simulink model "MdXXHolderChk"  (R2024b)
settings: Solver=FixedStepDiscrete  StartTime=0.0  StopTime=10.0  FixedStep=0.01  RelTol=1e-3
undefined symbols (not defined in the file or in its folder): KeSMSwAcsMd32SecRwLtStBkReclnUpwdDnwdPos1_Val, KeSMSwAcsMd53SecRwRtStBkReclnUpwdDnwdPos1_Val, SeatChldLkSt
libraries: simulink x41
(part 3 of 5)

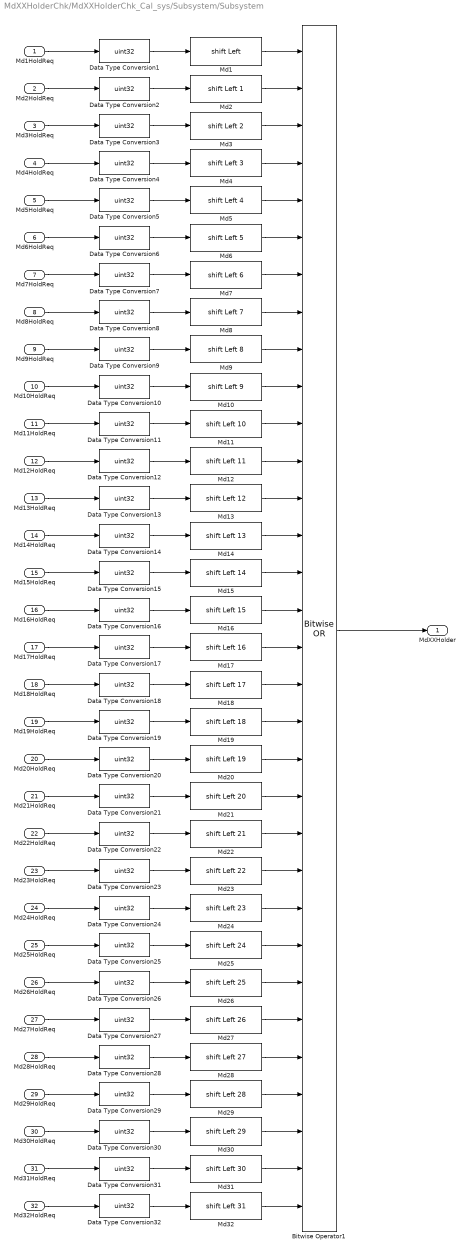
== system MdXXHolderChk/MdXXHolderChk_Cal_sys/Subsystem/Subsystem ==
  Md1HoldReq : Inport
  Md2HoldReq : Inport  Port=2
  Md3HoldReq : Inport  Port=3
  Md4HoldReq : Inport  Port=4
  Md5HoldReq : Inport  Port=5
  Md6HoldReq : Inport  Port=6
  Md7HoldReq : Inport  Port=7
  Md8HoldReq : Inport  Port=8
  Md9HoldReq : Inport  Port=9
  Md10HoldReq : Inport  Port=10
  Md11HoldReq : Inport  Port=11
  Md12HoldReq : Inport  Port=12
  Md13HoldReq : Inport  Port=13
  Md14HoldReq : Inport  Port=14
  Md15HoldReq : Inport  Port=15
  Md16HoldReq : Inport  Port=16
  Md17HoldReq : Inport  Port=17
  Md18HoldReq : Inport  Port=18
  Md19HoldReq : Inport  Port=19
  Md20HoldReq : Inport  Port=20
  Md21HoldReq : Inport  Port=21
  Md22HoldReq : Inport  Port=22
  Md23HoldReq : Inport  Port=23
  Md24HoldReq : Inport  Port=24
  Md25HoldReq : Inport  Port=25
  Md26HoldReq : Inport  Port=26
  Md27HoldReq : Inport  Port=27
  Md28HoldReq : Inport  Port=28
  Md29HoldReq : Inport  Port=29
  Md30HoldReq : Inport  Port=30
  Md31HoldReq : Inport  Port=31
  Md32HoldReq : Inport  Port=32
  Bitwise Operator1 : simulink/Logic and Bit Operations/Bitwise Operator  logicop=OR  UseBitMask=off  NumInputPorts=32  BitMask=bin2dec('11011001')  BitMaskRealWorld=Stored Integer
  Data Type Conversion{1..32} (32 alike) : DataTypeConversion  OutDataTypeStr=uint32  SaturateOnIntegerOverflow=off  RndMeth=Floor
  Md1 : ArithShift  BitShiftDirection=Left
  Md10 : ArithShift  BitShiftNumber=9  BitShiftDirection=Left
  Md11 : ArithShift  BitShiftNumber=10  BitShiftDirection=Left
  Md12 : ArithShift  BitShiftNumber=11  BitShiftDirection=Left
  Md13 : ArithShift  BitShiftNumber=12  BitShiftDirection=Left
  Md14 : ArithShift  BitShiftNumber=13  BitShiftDirection=Left
  Md15 : ArithShift  BitShiftNumber=14  BitShiftDirection=Left
  Md16 : ArithShift  BitShiftNumber=15  BitShiftDirection=Left
  Md17 : ArithShift  BitShiftNumber=16  BitShiftDirection=Left
  Md18 : ArithShift  BitShiftNumber=17  BitShiftDirection=Left
  Md19 : ArithShift  BitShiftNumber=18  BitShiftDirection=Left
  Md2 : ArithShift  BitShiftNumber=1  BitShiftDirection=Left
  Md20 : ArithShift  BitShiftNumber=19  BitShiftDirection=Left
  Md21 : ArithShift  BitShiftNumber=20  BitShiftDirection=Left
  Md22 : ArithShift  BitShiftNumber=21  BitShiftDirection=Left
  Md23 : ArithShift  BitShiftNumber=22  BitShiftDirection=Left
  Md24 : ArithShift  BitShiftNumber=23  BitShiftDirection=Left
  Md25 : ArithShift  BitShiftNumber=24  BitShiftDirection=Left
  Md26 : ArithShift  BitShiftNumber=25  BitShiftDirection=Left
  Md27 : ArithShift  BitShiftNumber=26  BitShiftDirection=Left
  Md28 : ArithShift  BitShiftNumber=27  BitShiftDirection=Left
  Md29 : ArithShift  BitShiftNumber=28  BitShiftDirection=Left
  Md3 : ArithShift  BitShiftNumber=2  BitShiftDirection=Left
  Md30 : ArithShift  BitShiftNumber=29  BitShiftDirection=Left
  Md31 : ArithShift  BitShiftNumber=30  BitShiftDirection=Left
  Md32 : ArithShift  BitShiftNumber=31  BitShiftDirection=Left
  Md4 : ArithShift  BitShiftNumber=3  BitShiftDirection=Left
  Md5 : ArithShift  BitShiftNumber=4  BitShiftDirection=Left
  Md6 : ArithShift  BitShiftNumber=5  BitShiftDirection=Left
  Md7 : ArithShift  BitShiftNumber=6  BitShiftDirection=Left
  Md8 : ArithShift  BitShiftNumber=7  BitShiftDirection=Left
  Md9 : ArithShift  BitShiftNumber=8  BitShiftDirection=Left
  MdXXHolder : Outport  VectorParamsAs1DForOutWhenUnconnected=off
  wires:
  Md30HoldReq/1 -> Data Type Conversion30/1
  Md3/1 -> Bitwise Operator1/3
  Data Type Conversion9/1 -> Md9/1
  Md5HoldReq/1 -> Data Type Conversion5/1
  Md13HoldReq/1 -> Data Type Conversion13/1
  Data Type Conversion32/1 -> Md32/1
  Md15HoldReq/1 -> Data Type Conversion15/1
  Data Type Conversion8/1 -> Md8/1
  Data Type Conversion3/1 -> Md3/1
  Md7HoldReq/1 -> Data Type Conversion7/1
  Md12HoldReq/1 -> Data Type Conversion12/1
  Data Type Conversion21/1 -> Md21/1
  Data Type Conversion12/1 -> Md12/1
  Md10HoldReq/1 -> Data Type Conversion10/1
  Md5/1 -> Bitwise Operator1/5
  Md14/1 -> Bitwise Operator1/14
  Md1/1 -> Bitwise Operator1/1
  Md9HoldReq/1 -> Data Type Conversion9/1
  Data Type Conversion27/1 -> Md27/1
  Data Type Conversion15/1 -> Md15/1
  Md29/1 -> Bitwise Operator1/29
  Md23/1 -> Bitwise Operator1/23
  Data Type Conversion10/1 -> Md10/1
  Md12/1 -> Bitwise Operator1/12
  Md31HoldReq/1 -> Data Type Conversion31/1
  Data Type Conversion22/1 -> Md22/1
  Bitwise Operator1/1 -> MdXXHolder/1
  Data Type Conversion31/1 -> Md31/1
  Md4/1 -> Bitwise Operator1/4
  Md27/1 -> Bitwise Operator1/27
  Data Type Conversion18/1 -> Md18/1
  Md9/1 -> Bitwise Operator1/9
  Md3HoldReq/1 -> Data Type Conversion3/1
  Data Type Conversion25/1 -> Md25/1
  Md14HoldReq/1 -> Data Type Conversion14/1
  Md27HoldReq/1 -> Data Type Conversion27/1
  Md4HoldReq/1 -> Data Type Conversion4/1
  Md7/1 -> Bitwise Operator1/7
  Md18HoldReq/1 -> Data Type Conversion18/1
  Md8/1 -> Bitwise Operator1/8
  Data Type Conversion7/1 -> Md7/1
  Data Type Conversion26/1 -> Md26/1
  Md17/1 -> Bitwise Operator1/17
  Data Type Conversion4/1 -> Md4/1
  Md18/1 -> Bitwise Operator1/18
  Md22HoldReq/1 -> Data Type Conversion22/1
  Md13/1 -> Bitwise Operator1/13
  Md2HoldReq/1 -> Data Type Conversion2/1
  Data Type Conversion2/1 -> Md2/1
  Md1HoldReq/1 -> Data Type Conversion1/1
  Data Type Conversion24/1 -> Md24/1
  Data Type Conversion13/1 -> Md13/1
  Md24HoldReq/1 -> Data Type Conversion24/1
  Data Type Conversion14/1 -> Md14/1
  Md22/1 -> Bitwise Operator1/22
  Data Type Conversion30/1 -> Md30/1
  Md32HoldReq/1 -> Data Type Conversion32/1
  Data Type Conversion5/1 -> Md5/1
  Md20HoldReq/1 -> Data Type Conversion20/1
  Md10/1 -> Bitwise Operator1/10
  Md11/1 -> Bitwise Operator1/11
  Data Type Conversion20/1 -> Md20/1
  Md21HoldReq/1 -> Data Type Conversion21/1
  Data Type Conversion23/1 -> Md23/1
  Md23HoldReq/1 -> Data Type Conversion23/1
  Md25HoldReq/1 -> Data Type Conversion25/1
  Data Type Conversion17/1 -> Md17/1
  Md17HoldReq/1 -> Data Type Conversion17/1
  Md6/1 -> Bitwise Operator1/6
  Md16/1 -> Bitwise Operator1/16
  Md15/1 -> Bitwise Operator1/15
  Md19/1 -> Bitwise Operator1/19
  Md6HoldReq/1 -> Data Type Conversion6/1
  Data Type Conversion19/1 -> Md19/1
  Md20/1 -> Bitwise Operator1/20
  Md21/1 -> Bitwise Operator1/21
  Md24/1 -> Bitwise Operator1/24
  Md25/1 -> Bitwise Operator1/25
  Md26/1 -> Bitwise Operator1/26
  Md28/1 -> Bitwise Operator1/28
  Md30/1 -> Bitwise Operator1/30
  Md31/1 -> Bitwise Operator1/31
  Md32/1 -> Bitwise Operator1/32
  Md2/1 -> Bitwise Operator1/2
  Md11HoldReq/1 -> Data Type Conversion11/1
  Data Type Conversion11/1 -> Md11/1
  Data Type Conversion6/1 -> Md6/1
  Md28HoldReq/1 -> Data Type Conversion28/1
  Data Type Conversion28/1 -> Md28/1
  Md16HoldReq/1 -> Data Type Conversion16/1
  Data Type Conversion16/1 -> Md16/1
  Md26HoldReq/1 -> Data Type Conversion26/1
  Md19HoldReq/1 -> Data Type Conversion19/1
  Data Type Conversion1/1 -> Md1/1
  Md8HoldReq/1 -> Data Type Conversion8/1
  Data Type Conversion29/1 -> Md29/1
  Md29HoldReq/1 -> Data Type Conversion29/1

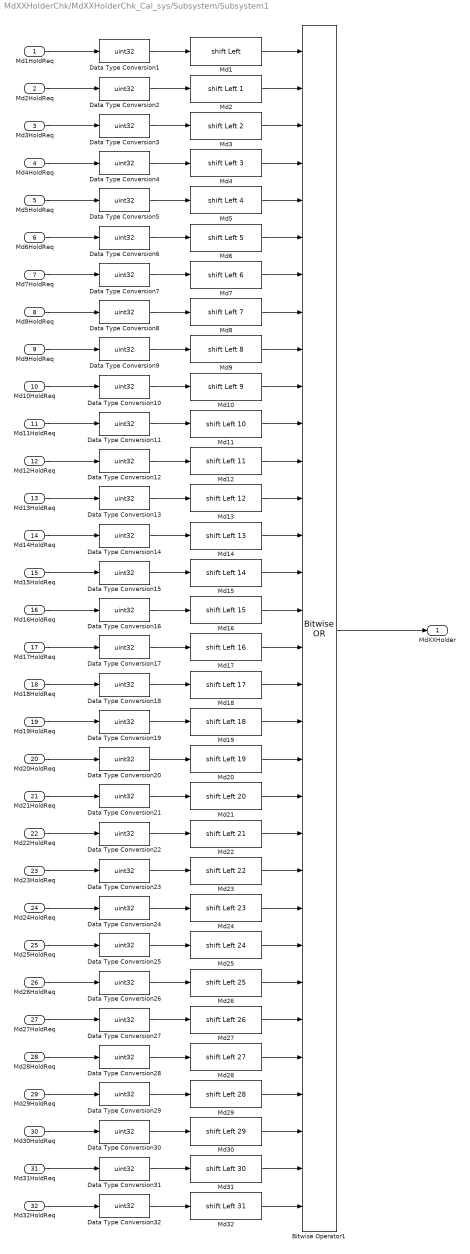
== system MdXXHolderChk/MdXXHolderChk_Cal_sys/Subsystem/Subsystem1 ==
  Md1HoldReq : Inport
  Md2HoldReq : Inport  Port=2
  Md3HoldReq : Inport  Port=3
  Md4HoldReq : Inport  Port=4
  Md5HoldReq : Inport  Port=5
  Md6HoldReq : Inport  Port=6
  Md7HoldReq : Inport  Port=7
  Md8HoldReq : Inport  Port=8
  Md9HoldReq : Inport  Port=9
  Md10HoldReq : Inport  Port=10
  Md11HoldReq : Inport  Port=11
  Md12HoldReq : Inport  Port=12
  Md13HoldReq : Inport  Port=13
  Md14HoldReq : Inport  Port=14
  Md15HoldReq : Inport  Port=15
  Md16HoldReq : Inport  Port=16
  Md17HoldReq : Inport  Port=17
  Md18HoldReq : Inport  Port=18
  Md19HoldReq : Inport  Port=19
  Md20HoldReq : Inport  Port=20
  Md21HoldReq : Inport  Port=21
  Md22HoldReq : Inport  Port=22
  Md23HoldReq : Inport  Port=23
  Md24HoldReq : Inport  Port=24
  Md25HoldReq : Inport  Port=25
  Md26HoldReq : Inport  Port=26
  Md27HoldReq : Inport  Port=27
  Md28HoldReq : Inport  Port=28
  Md29HoldReq : Inport  Port=29
  Md30HoldReq : Inport  Port=30
  Md31HoldReq : Inport  Port=31
  Md32HoldReq : Inport  Port=32
  Bitwise Operator1 : simulink/Logic and Bit Operations/Bitwise Operator  logicop=OR  UseBitMask=off  NumInputPorts=32  BitMask=bin2dec('11011001')  BitMaskRealWorld=Stored Integer
  Data Type Conversion{1..32} (32 alike) : DataTypeConversion  OutDataTypeStr=uint32  SaturateOnIntegerOverflow=off  RndMeth=Floor
  Md1 : ArithShift  BitShiftDirection=Left
  Md10 : ArithShift  BitShiftNumber=9  BitShiftDirection=Left
  Md11 : ArithShift  BitShiftNumber=10  BitShiftDirection=Left
  Md12 : ArithShift  BitShiftNumber=11  BitShiftDirection=Left
  Md13 : ArithShift  BitShiftNumber=12  BitShiftDirection=Left
  Md14 : ArithShift  BitShiftNumber=13  BitShiftDirection=Left
  Md15 : ArithShift  BitShiftNumber=14  BitShiftDirection=Left
  Md16 : ArithShift  BitShiftNumber=15  BitShiftDirection=Left
  Md17 : ArithShift  BitShiftNumber=16  BitShiftDirection=Left
  Md18 : ArithShift  BitShiftNumber=17  BitShiftDirection=Left
  Md19 : ArithShift  BitShiftNumber=18  BitShiftDirection=Left
  Md2 : ArithShift  BitShiftNumber=1  BitShiftDirection=Left
  Md20 : ArithShift  BitShiftNumber=19  BitShiftDirection=Left
  Md21 : ArithShift  BitShiftNumber=20  BitShiftDirection=Left
  Md22 : ArithShift  BitShiftNumber=21  BitShiftDirection=Left
  Md23 : ArithShift  BitShiftNumber=22  BitShiftDirection=Left
  Md24 : ArithShift  BitShiftNumber=23  BitShiftDirection=Left
  Md25 : ArithShift  BitShiftNumber=24  BitShiftDirection=Left
  Md26 : ArithShift  BitShiftNumber=25  BitShiftDirection=Left
  Md27 : ArithShift  BitShiftNumber=26  BitShiftDirection=Left
  Md28 : ArithShift  BitShiftNumber=27  BitShiftDirection=Left
  Md29 : ArithShift  BitShiftNumber=28  BitShiftDirection=Left
  Md3 : ArithShift  BitShiftNumber=2  BitShiftDirection=Left
  Md30 : ArithShift  BitShiftNumber=29  BitShiftDirection=Left
  Md31 : ArithShift  BitShiftNumber=30  BitShiftDirection=Left
  Md32 : ArithShift  BitShiftNumber=31  BitShiftDirection=Left
  Md4 : ArithShift  BitShiftNumber=3  BitShiftDirection=Left
  Md5 : ArithShift  BitShiftNumber=4  BitShiftDirection=Left
  Md6 : ArithShift  BitShiftNumber=5  BitShiftDirection=Left
  Md7 : ArithShift  BitShiftNumber=6  BitShiftDirection=Left
  Md8 : ArithShift  BitShiftNumber=7  BitShiftDirection=Left
  Md9 : ArithShift  BitShiftNumber=8  BitShiftDirection=Left
  MdXXHolder : Outport  VectorParamsAs1DForOutWhenUnconnected=off
  wires:
  Md30HoldReq/1 -> Data Type Conversion30/1
  Md3/1 -> Bitwise Operator1/3
  Data Type Conversion9/1 -> Md9/1
  Md5HoldReq/1 -> Data Type Conversion5/1
  Md13HoldReq/1 -> Data Type Conversion13/1
  Data Type Conversion32/1 -> Md32/1
  Md15HoldReq/1 -> Data Type Conversion15/1
  Data Type Conversion8/1 -> Md8/1
  Data Type Conversion3/1 -> Md3/1
  Md7HoldReq/1 -> Data Type Conversion7/1
  Md12HoldReq/1 -> Data Type Conversion12/1
  Data Type Conversion21/1 -> Md21/1
  Data Type Conversion12/1 -> Md12/1
  Md10HoldReq/1 -> Data Type Conversion10/1
  Md5/1 -> Bitwise Operator1/5
  Md14/1 -> Bitwise Operator1/14
  Md1/1 -> Bitwise Operator1/1
  Md9HoldReq/1 -> Data Type Conversion9/1
  Data Type Conversion27/1 -> Md27/1
  Data Type Conversion15/1 -> Md15/1
  Md29/1 -> Bitwise Operator1/29
  Md23/1 -> Bitwise Operator1/23
  Data Type Conversion10/1 -> Md10/1
  Md12/1 -> Bitwise Operator1/12
  Md31HoldReq/1 -> Data Type Conversion31/1
  Data Type Conversion22/1 -> Md22/1
  Bitwise Operator1/1 -> MdXXHolder/1
  Data Type Conversion31/1 -> Md31/1
  Md4/1 -> Bitwise Operator1/4
  Md27/1 -> Bitwise Operator1/27
  Data Type Conversion18/1 -> Md18/1
  Md9/1 -> Bitwise Operator1/9
  Md3HoldReq/1 -> Data Type Conversion3/1
  Data Type Conversion25/1 -> Md25/1
  Md14HoldReq/1 -> Data Type Conversion14/1
  Md27HoldReq/1 -> Data Type Conversion27/1
  Md4HoldReq/1 -> Data Type Conversion4/1
  Md7/1 -> Bitwise Operator1/7
  Md18HoldReq/1 -> Data Type Conversion18/1
  Md8/1 -> Bitwise Operator1/8
  Data Type Conversion7/1 -> Md7/1
  Data Type Conversion26/1 -> Md26/1
  Md17/1 -> Bitwise Operator1/17
  Data Type Conversion4/1 -> Md4/1
  Md18/1 -> Bitwise Operator1/18
  Md22HoldReq/1 -> Data Type Conversion22/1
  Md13/1 -> Bitwise Operator1/13
  Md2HoldReq/1 -> Data Type Conversion2/1
  Data Type Conversion2/1 -> Md2/1
  Md1HoldReq/1 -> Data Type Conversion1/1
  Data Type Conversion24/1 -> Md24/1
  Data Type Conversion13/1 -> Md13/1
  Md24HoldReq/1 -> Data Type Conversion24/1
  Data Type Conversion14/1 -> Md14/1
  Md22/1 -> Bitwise Operator1/22
  Data Type Conversion30/1 -> Md30/1
  Md32HoldReq/1 -> Data Type Conversion32/1
  Data Type Conversion5/1 -> Md5/1
  Md20HoldReq/1 -> Data Type Conversion20/1
  Md10/1 -> Bitwise Operator1/10
  Md11/1 -> Bitwise Operator1/11
  Data Type Conversion20/1 -> Md20/1
  Md21HoldReq/1 -> Data Type Conversion21/1
  Data Type Conversion23/1 -> Md23/1
  Md23HoldReq/1 -> Data Type Conversion23/1
  Md25HoldReq/1 -> Data Type Conversion25/1
  Data Type Conversion17/1 -> Md17/1
  Md17HoldReq/1 -> Data Type Conversion17/1
  Md6/1 -> Bitwise Operator1/6
  Md16/1 -> Bitwise Operator1/16
  Md15/1 -> Bitwise Operator1/15
  Md19/1 -> Bitwise Operator1/19
  Md6HoldReq/1 -> Data Type Conversion6/1
  Data Type Conversion19/1 -> Md19/1
  Md20/1 -> Bitwise Operator1/20
  Md21/1 -> Bitwise Operator1/21
  Md24/1 -> Bitwise Operator1/24
  Md25/1 -> Bitwise Operator1/25
  Md26/1 -> Bitwise Operator1/26
  Md28/1 -> Bitwise Operator1/28
  Md30/1 -> Bitwise Operator1/30
  Md31/1 -> Bitwise Operator1/31
  Md32/1 -> Bitwise Operator1/32
  Md2/1 -> Bitwise Operator1/2
  Md11HoldReq/1 -> Data Type Conversion11/1
  Data Type Conversion11/1 -> Md11/1
  Data Type Conversion6/1 -> Md6/1
  Md28HoldReq/1 -> Data Type Conversion28/1
  Data Type Conversion28/1 -> Md28/1
  Md16HoldReq/1 -> Data Type Conversion16/1
  Data Type Conversion16/1 -> Md16/1
  Md26HoldReq/1 -> Data Type Conversion26/1
  Md19HoldReq/1 -> Data Type Conversion19/1
  Data Type Conversion1/1 -> Md1/1
  Md8HoldReq/1 -> Data Type Conversion8/1
  Data Type Conversion29/1 -> Md29/1
  Md29HoldReq/1 -> Data Type Conversion29/1

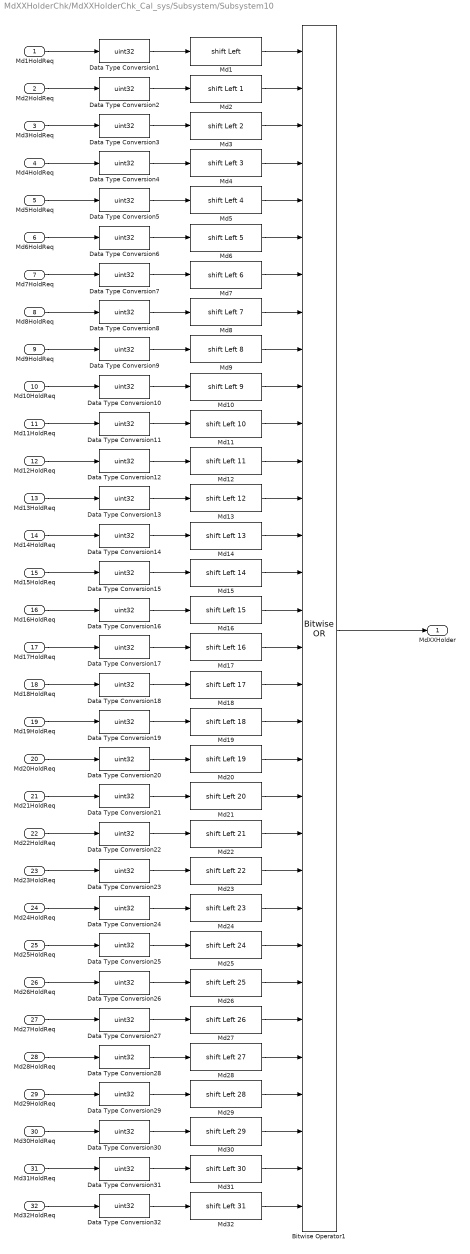
== system MdXXHolderChk/MdXXHolderChk_Cal_sys/Subsystem/Subsystem10 ==
  Md1HoldReq : Inport
  Md2HoldReq : Inport  Port=2
  Md3HoldReq : Inport  Port=3
  Md4HoldReq : Inport  Port=4
  Md5HoldReq : Inport  Port=5
  Md6HoldReq : Inport  Port=6
  Md7HoldReq : Inport  Port=7
  Md8HoldReq : Inport  Port=8
  Md9HoldReq : Inport  Port=9
  Md10HoldReq : Inport  Port=10
  Md11HoldReq : Inport  Port=11
  Md12HoldReq : Inport  Port=12
  Md13HoldReq : Inport  Port=13
  Md14HoldReq : Inport  Port=14
  Md15HoldReq : Inport  Port=15
  Md16HoldReq : Inport  Port=16
  Md17HoldReq : Inport  Port=17
  Md18HoldReq : Inport  Port=18
  Md19HoldReq : Inport  Port=19
  Md20HoldReq : Inport  Port=20
  Md21HoldReq : Inport  Port=21
  Md22HoldReq : Inport  Port=22
  Md23HoldReq : Inport  Port=23
  Md24HoldReq : Inport  Port=24
  Md25HoldReq : Inport  Port=25
  Md26HoldReq : Inport  Port=26
  Md27HoldReq : Inport  Port=27
  Md28HoldReq : Inport  Port=28
  Md29HoldReq : Inport  Port=29
  Md30HoldReq : Inport  Port=30
  Md31HoldReq : Inport  Port=31
  Md32HoldReq : Inport  Port=32
  Bitwise Operator1 : simulink/Logic and Bit Operations/Bitwise Operator  logicop=OR  UseBitMask=off  NumInputPorts=32  BitMask=bin2dec('11011001')  BitMaskRealWorld=Stored Integer
  Data Type Conversion{1..32} (32 alike) : DataTypeConversion  OutDataTypeStr=uint32  SaturateOnIntegerOverflow=off  RndMeth=Floor
  Md1 : ArithShift  BitShiftDirection=Left
  Md10 : ArithShift  BitShiftNumber=9  BitShiftDirection=Left
  Md11 : ArithShift  BitShiftNumber=10  BitShiftDirection=Left
  Md12 : ArithShift  BitShiftNumber=11  BitShiftDirection=Left
  Md13 : ArithShift  BitShiftNumber=12  BitShiftDirection=Left
  Md14 : ArithShift  BitShiftNumber=13  BitShiftDirection=Left
  Md15 : ArithShift  BitShiftNumber=14  BitShiftDirection=Left
  Md16 : ArithShift  BitShiftNumber=15  BitShiftDirection=Left
  Md17 : ArithShift  BitShiftNumber=16  BitShiftDirection=Left
  Md18 : ArithShift  BitShiftNumber=17  BitShiftDirection=Left
  Md19 : ArithShift  BitShiftNumber=18  BitShiftDirection=Left
  Md2 : ArithShift  BitShiftNumber=1  BitShiftDirection=Left
  Md20 : ArithShift  BitShiftNumber=19  BitShiftDirection=Left
  Md21 : ArithShift  BitShiftNumber=20  BitShiftDirection=Left
  Md22 : ArithShift  BitShiftNumber=21  BitShiftDirection=Left
  Md23 : ArithShift  BitShiftNumber=22  BitShiftDirection=Left
  Md24 : ArithShift  BitShiftNumber=23  BitShiftDirection=Left
  Md25 : ArithShift  BitShiftNumber=24  BitShiftDirection=Left
  Md26 : ArithShift  BitShiftNumber=25  BitShiftDirection=Left
  Md27 : ArithShift  BitShiftNumber=26  BitShiftDirection=Left
  Md28 : ArithShift  BitShiftNumber=27  BitShiftDirection=Left
  Md29 : ArithShift  BitShiftNumber=28  BitShiftDirection=Left
  Md3 : ArithShift  BitShiftNumber=2  BitShiftDirection=Left
  Md30 : ArithShift  BitShiftNumber=29  BitShiftDirection=Left
  Md31 : ArithShift  BitShiftNumber=30  BitShiftDirection=Left
  Md32 : ArithShift  BitShiftNumber=31  BitShiftDirection=Left
  Md4 : ArithShift  BitShiftNumber=3  BitShiftDirection=Left
  Md5 : ArithShift  BitShiftNumber=4  BitShiftDirection=Left
  Md6 : ArithShift  BitShiftNumber=5  BitShiftDirection=Left
  Md7 : ArithShift  BitShiftNumber=6  BitShiftDirection=Left
  Md8 : ArithShift  BitShiftNumber=7  BitShiftDirection=Left
  Md9 : ArithShift  BitShiftNumber=8  BitShiftDirection=Left
  MdXXHolder : Outport  VectorParamsAs1DForOutWhenUnconnected=off
  wires:
  Md30HoldReq/1 -> Data Type Conversion30/1
  Md3/1 -> Bitwise Operator1/3
  Data Type Conversion9/1 -> Md9/1
  Md5HoldReq/1 -> Data Type Conversion5/1
  Md13HoldReq/1 -> Data Type Conversion13/1
  Data Type Conversion32/1 -> Md32/1
  Md15HoldReq/1 -> Data Type Conversion15/1
  Data Type Conversion8/1 -> Md8/1
  Data Type Conversion3/1 -> Md3/1
  Md7HoldReq/1 -> Data Type Conversion7/1
  Md12HoldReq/1 -> Data Type Conversion12/1
  Data Type Conversion21/1 -> Md21/1
  Data Type Conversion12/1 -> Md12/1
  Md10HoldReq/1 -> Data Type Conversion10/1
  Md5/1 -> Bitwise Operator1/5
  Md14/1 -> Bitwise Operator1/14
  Md1/1 -> Bitwise Operator1/1
  Md9HoldReq/1 -> Data Type Conversion9/1
  Data Type Conversion27/1 -> Md27/1
  Data Type Conversion15/1 -> Md15/1
  Md29/1 -> Bitwise Operator1/29
  Md23/1 -> Bitwise Operator1/23
  Data Type Conversion10/1 -> Md10/1
  Md12/1 -> Bitwise Operator1/12
  Md31HoldReq/1 -> Data Type Conversion31/1
  Data Type Conversion22/1 -> Md22/1
  Bitwise Operator1/1 -> MdXXHolder/1
  Data Type Conversion31/1 -> Md31/1
  Md4/1 -> Bitwise Operator1/4
  Md27/1 -> Bitwise Operator1/27
  Data Type Conversion18/1 -> Md18/1
  Md9/1 -> Bitwise Operator1/9
  Md3HoldReq/1 -> Data Type Conversion3/1
  Data Type Conversion25/1 -> Md25/1
  Md14HoldReq/1 -> Data Type Conversion14/1
  Md27HoldReq/1 -> Data Type Conversion27/1
  Md4HoldReq/1 -> Data Type Conversion4/1
  Md7/1 -> Bitwise Operator1/7
  Md18HoldReq/1 -> Data Type Conversion18/1
  Md8/1 -> Bitwise Operator1/8
  Data Type Conversion7/1 -> Md7/1
  Data Type Conversion26/1 -> Md26/1
  Md17/1 -> Bitwise Operator1/17
  Data Type Conversion4/1 -> Md4/1
  Md18/1 -> Bitwise Operator1/18
  Md22HoldReq/1 -> Data Type Conversion22/1
  Md13/1 -> Bitwise Operator1/13
  Md2HoldReq/1 -> Data Type Conversion2/1
  Data Type Conversion2/1 -> Md2/1
  Md1HoldReq/1 -> Data Type Conversion1/1
  Data Type Conversion24/1 -> Md24/1
  Data Type Conversion13/1 -> Md13/1
  Md24HoldReq/1 -> Data Type Conversion24/1
  Data Type Conversion14/1 -> Md14/1
  Md22/1 -> Bitwise Operator1/22
  Data Type Conversion30/1 -> Md30/1
  Md32HoldReq/1 -> Data Type Conversion32/1
  Data Type Conversion5/1 -> Md5/1
  Md20HoldReq/1 -> Data Type Conversion20/1
  Md10/1 -> Bitwise Operator1/10
  Md11/1 -> Bitwise Operator1/11
  Data Type Conversion20/1 -> Md20/1
  Md21HoldReq/1 -> Data Type Conversion21/1
  Data Type Conversion23/1 -> Md23/1
  Md23HoldReq/1 -> Data Type Conversion23/1
  Md25HoldReq/1 -> Data Type Conversion25/1
  Data Type Conversion17/1 -> Md17/1
  Md17HoldReq/1 -> Data Type Conversion17/1
  Md6/1 -> Bitwise Operator1/6
  Md16/1 -> Bitwise Operator1/16
  Md15/1 -> Bitwise Operator1/15
  Md19/1 -> Bitwise Operator1/19
  Md6HoldReq/1 -> Data Type Conversion6/1
  Data Type Conversion19/1 -> Md19/1
  Md20/1 -> Bitwise Operator1/20
  Md21/1 -> Bitwise Operator1/21
  Md24/1 -> Bitwise Operator1/24
  Md25/1 -> Bitwise Operator1/25
  Md26/1 -> Bitwise Operator1/26
  Md28/1 -> Bitwise Operator1/28
  Md30/1 -> Bitwise Operator1/30
  Md31/1 -> Bitwise Operator1/31
  Md32/1 -> Bitwise Operator1/32
  Md2/1 -> Bitwise Operator1/2
  Md11HoldReq/1 -> Data Type Conversion11/1
  Data Type Conversion11/1 -> Md11/1
  Data Type Conversion6/1 -> Md6/1
  Md28HoldReq/1 -> Data Type Conversion28/1
  Data Type Conversion28/1 -> Md28/1
  Md16HoldReq/1 -> Data Type Conversion16/1
  Data Type Conversion16/1 -> Md16/1
  Md26HoldReq/1 -> Data Type Conversion26/1
  Md19HoldReq/1 -> Data Type Conversion19/1
  Data Type Conversion1/1 -> Md1/1
  Md8HoldReq/1 -> Data Type Conversion8/1
  Data Type Conversion29/1 -> Md29/1
  Md29HoldReq/1 -> Data Type Conversion29/1

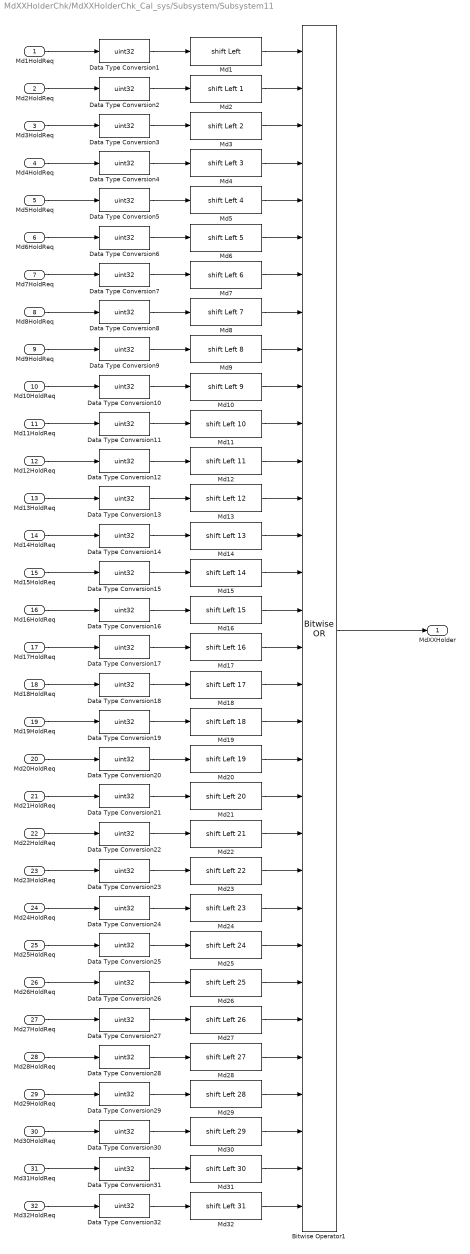
== system MdXXHolderChk/MdXXHolderChk_Cal_sys/Subsystem/Subsystem11 ==
  Md1HoldReq : Inport
  Md2HoldReq : Inport  Port=2
  Md3HoldReq : Inport  Port=3
  Md4HoldReq : Inport  Port=4
  Md5HoldReq : Inport  Port=5
  Md6HoldReq : Inport  Port=6
  Md7HoldReq : Inport  Port=7
  Md8HoldReq : Inport  Port=8
  Md9HoldReq : Inport  Port=9
  Md10HoldReq : Inport  Port=10
  Md11HoldReq : Inport  Port=11
  Md12HoldReq : Inport  Port=12
  Md13HoldReq : Inport  Port=13
  Md14HoldReq : Inport  Port=14
  Md15HoldReq : Inport  Port=15
  Md16HoldReq : Inport  Port=16
  Md17HoldReq : Inport  Port=17
  Md18HoldReq : Inport  Port=18
  Md19HoldReq : Inport  Port=19
  Md20HoldReq : Inport  Port=20
  Md21HoldReq : Inport  Port=21
  Md22HoldReq : Inport  Port=22
  Md23HoldReq : Inport  Port=23
  Md24HoldReq : Inport  Port=24
  Md25HoldReq : Inport  Port=25
  Md26HoldReq : Inport  Port=26
  Md27HoldReq : Inport  Port=27
  Md28HoldReq : Inport  Port=28
  Md29HoldReq : Inport  Port=29
  Md30HoldReq : Inport  Port=30
  Md31HoldReq : Inport  Port=31
  Md32HoldReq : Inport  Port=32
  Bitwise Operator1 : simulink/Logic and Bit Operations/Bitwise Operator  logicop=OR  UseBitMask=off  NumInputPorts=32  BitMask=bin2dec('11011001')  BitMaskRealWorld=Stored Integer
  Data Type Conversion{1..32} (32 alike) : DataTypeConversion  OutDataTypeStr=uint32  SaturateOnIntegerOverflow=off  RndMeth=Floor
  Md1 : ArithShift  BitShiftDirection=Left
  Md10 : ArithShift  BitShiftNumber=9  BitShiftDirection=Left
  Md11 : ArithShift  BitShiftNumber=10  BitShiftDirection=Left
  Md12 : ArithShift  BitShiftNumber=11  BitShiftDirection=Left
  Md13 : ArithShift  BitShiftNumber=12  BitShiftDirection=Left
  Md14 : ArithShift  BitShiftNumber=13  BitShiftDirection=Left
  Md15 : ArithShift  BitShiftNumber=14  BitShiftDirection=Left
  Md16 : ArithShift  BitShiftNumber=15  BitShiftDirection=Left
  Md17 : ArithShift  BitShiftNumber=16  BitShiftDirection=Left
  Md18 : ArithShift  BitShiftNumber=17  BitShiftDirection=Left
  Md19 : ArithShift  BitShiftNumber=18  BitShiftDirection=Left
  Md2 : ArithShift  BitShiftNumber=1  BitShiftDirection=Left
  Md20 : ArithShift  BitShiftNumber=19  BitShiftDirection=Left
  Md21 : ArithShift  BitShiftNumber=20  BitShiftDirection=Left
  Md22 : ArithShift  BitShiftNumber=21  BitShiftDirection=Left
  Md23 : ArithShift  BitShiftNumber=22  BitShiftDirection=Left
  Md24 : ArithShift  BitShiftNumber=23  BitShiftDirection=Left
  Md25 : ArithShift  BitShiftNumber=24  BitShiftDirection=Left
  Md26 : ArithShift  BitShiftNumber=25  BitShiftDirection=Left
  Md27 : ArithShift  BitShiftNumber=26  BitShiftDirection=Left
  Md28 : ArithShift  BitShiftNumber=27  BitShiftDirection=Left
  Md29 : ArithShift  BitShiftNumber=28  BitShiftDirection=Left
  Md3 : ArithShift  BitShiftNumber=2  BitShiftDirection=Left
  Md30 : ArithShift  BitShiftNumber=29  BitShiftDirection=Left
  Md31 : ArithShift  BitShiftNumber=30  BitShiftDirection=Left
  Md32 : ArithShift  BitShiftNumber=31  BitShiftDirection=Left
  Md4 : ArithShift  BitShiftNumber=3  BitShiftDirection=Left
  Md5 : ArithShift  BitShiftNumber=4  BitShiftDirection=Left
  Md6 : ArithShift  BitShiftNumber=5  BitShiftDirection=Left
  Md7 : ArithShift  BitShiftNumber=6  BitShiftDirection=Left
  Md8 : ArithShift  BitShiftNumber=7  BitShiftDirection=Left
  Md9 : ArithShift  BitShiftNumber=8  BitShiftDirection=Left
  MdXXHolder : Outport  VectorParamsAs1DForOutWhenUnconnected=off
  wires:
  Md30HoldReq/1 -> Data Type Conversion30/1
  Md3/1 -> Bitwise Operator1/3
  Data Type Conversion9/1 -> Md9/1
  Md5HoldReq/1 -> Data Type Conversion5/1
  Md13HoldReq/1 -> Data Type Conversion13/1
  Data Type Conversion32/1 -> Md32/1
  Md15HoldReq/1 -> Data Type Conversion15/1
  Data Type Conversion8/1 -> Md8/1
  Data Type Conversion3/1 -> Md3/1
  Md7HoldReq/1 -> Data Type Conversion7/1
  Md12HoldReq/1 -> Data Type Conversion12/1
  Data Type Conversion21/1 -> Md21/1
  Data Type Conversion12/1 -> Md12/1
  Md10HoldReq/1 -> Data Type Conversion10/1
  Md5/1 -> Bitwise Operator1/5
  Md14/1 -> Bitwise Operator1/14
  Md1/1 -> Bitwise Operator1/1
  Md9HoldReq/1 -> Data Type Conversion9/1
  Data Type Conversion27/1 -> Md27/1
  Data Type Conversion15/1 -> Md15/1
  Md29/1 -> Bitwise Operator1/29
  Md23/1 -> Bitwise Operator1/23
  Data Type Conversion10/1 -> Md10/1
  Md12/1 -> Bitwise Operator1/12
  Md31HoldReq/1 -> Data Type Conversion31/1
  Data Type Conversion22/1 -> Md22/1
  Bitwise Operator1/1 -> MdXXHolder/1
  Data Type Conversion31/1 -> Md31/1
  Md4/1 -> Bitwise Operator1/4
  Md27/1 -> Bitwise Operator1/27
  Data Type Conversion18/1 -> Md18/1
  Md9/1 -> Bitwise Operator1/9
  Md3HoldReq/1 -> Data Type Conversion3/1
  Data Type Conversion25/1 -> Md25/1
  Md14HoldReq/1 -> Data Type Conversion14/1
  Md27HoldReq/1 -> Data Type Conversion27/1
  Md4HoldReq/1 -> Data Type Conversion4/1
  Md7/1 -> Bitwise Operator1/7
  Md18HoldReq/1 -> Data Type Conversion18/1
  Md8/1 -> Bitwise Operator1/8
  Data Type Conversion7/1 -> Md7/1
  Data Type Conversion26/1 -> Md26/1
  Md17/1 -> Bitwise Operator1/17
  Data Type Conversion4/1 -> Md4/1
  Md18/1 -> Bitwise Operator1/18
  Md22HoldReq/1 -> Data Type Conversion22/1
  Md13/1 -> Bitwise Operator1/13
  Md2HoldReq/1 -> Data Type Conversion2/1
  Data Type Conversion2/1 -> Md2/1
  Md1HoldReq/1 -> Data Type Conversion1/1
  Data Type Conversion24/1 -> Md24/1
  Data Type Conversion13/1 -> Md13/1
  Md24HoldReq/1 -> Data Type Conversion24/1
  Data Type Conversion14/1 -> Md14/1
  Md22/1 -> Bitwise Operator1/22
  Data Type Conversion30/1 -> Md30/1
  Md32HoldReq/1 -> Data Type Conversion32/1
  Data Type Conversion5/1 -> Md5/1
  Md20HoldReq/1 -> Data Type Conversion20/1
  Md10/1 -> Bitwise Operator1/10
  Md11/1 -> Bitwise Operator1/11
  Data Type Conversion20/1 -> Md20/1
  Md21HoldReq/1 -> Data Type Conversion21/1
  Data Type Conversion23/1 -> Md23/1
  Md23HoldReq/1 -> Data Type Conversion23/1
  Md25HoldReq/1 -> Data Type Conversion25/1
  Data Type Conversion17/1 -> Md17/1
  Md17HoldReq/1 -> Data Type Conversion17/1
  Md6/1 -> Bitwise Operator1/6
  Md16/1 -> Bitwise Operator1/16
  Md15/1 -> Bitwise Operator1/15
  Md19/1 -> Bitwise Operator1/19
  Md6HoldReq/1 -> Data Type Conversion6/1
  Data Type Conversion19/1 -> Md19/1
  Md20/1 -> Bitwise Operator1/20
  Md21/1 -> Bitwise Operator1/21
  Md24/1 -> Bitwise Operator1/24
  Md25/1 -> Bitwise Operator1/25
  Md26/1 -> Bitwise Operator1/26
  Md28/1 -> Bitwise Operator1/28
  Md30/1 -> Bitwise Operator1/30
  Md31/1 -> Bitwise Operator1/31
  Md32/1 -> Bitwise Operator1/32
  Md2/1 -> Bitwise Operator1/2
  Md11HoldReq/1 -> Data Type Conversion11/1
  Data Type Conversion11/1 -> Md11/1
  Data Type Conversion6/1 -> Md6/1
  Md28HoldReq/1 -> Data Type Conversion28/1
  Data Type Conversion28/1 -> Md28/1
  Md16HoldReq/1 -> Data Type Conversion16/1
  Data Type Conversion16/1 -> Md16/1
  Md26HoldReq/1 -> Data Type Conversion26/1
  Md19HoldReq/1 -> Data Type Conversion19/1
  Data Type Conversion1/1 -> Md1/1
  Md8HoldReq/1 -> Data Type Conversion8/1
  Data Type Conversion29/1 -> Md29/1
  Md29HoldReq/1 -> Data Type Conversion29/1

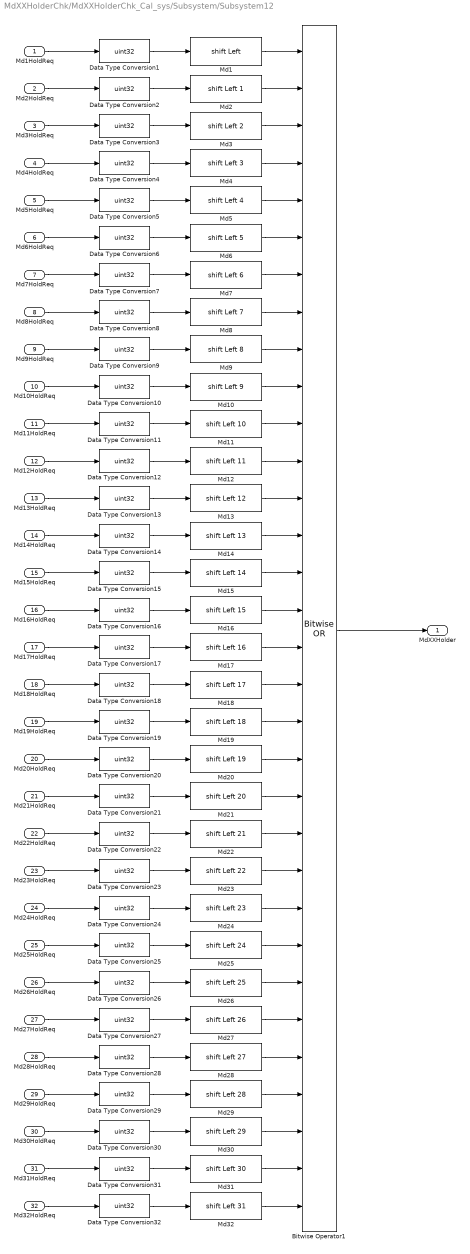
== system MdXXHolderChk/MdXXHolderChk_Cal_sys/Subsystem/Subsystem12 ==
  Md1HoldReq : Inport
  Md2HoldReq : Inport  Port=2
  Md3HoldReq : Inport  Port=3
  Md4HoldReq : Inport  Port=4
  Md5HoldReq : Inport  Port=5
  Md6HoldReq : Inport  Port=6
  Md7HoldReq : Inport  Port=7
  Md8HoldReq : Inport  Port=8
  Md9HoldReq : Inport  Port=9
  Md10HoldReq : Inport  Port=10
  Md11HoldReq : Inport  Port=11
  Md12HoldReq : Inport  Port=12
  Md13HoldReq : Inport  Port=13
  Md14HoldReq : Inport  Port=14
  Md15HoldReq : Inport  Port=15
  Md16HoldReq : Inport  Port=16
  Md17HoldReq : Inport  Port=17
  Md18HoldReq : Inport  Port=18
  Md19HoldReq : Inport  Port=19
  Md20HoldReq : Inport  Port=20
  Md21HoldReq : Inport  Port=21
  Md22HoldReq : Inport  Port=22
  Md23HoldReq : Inport  Port=23
  Md24HoldReq : Inport  Port=24
  Md25HoldReq : Inport  Port=25
  Md26HoldReq : Inport  Port=26
  Md27HoldReq : Inport  Port=27
  Md28HoldReq : Inport  Port=28
  Md29HoldReq : Inport  Port=29
  Md30HoldReq : Inport  Port=30
  Md31HoldReq : Inport  Port=31
  Md32HoldReq : Inport  Port=32
  Bitwise Operator1 : simulink/Logic and Bit Operations/Bitwise Operator  logicop=OR  UseBitMask=off  NumInputPorts=32  BitMask=bin2dec('11011001')  BitMaskRealWorld=Stored Integer
  Data Type Conversion{1..32} (32 alike) : DataTypeConversion  OutDataTypeStr=uint32  SaturateOnIntegerOverflow=off  RndMeth=Floor
  Md1 : ArithShift  BitShiftDirection=Left
  Md10 : ArithShift  BitShiftNumber=9  BitShiftDirection=Left
  Md11 : ArithShift  BitShiftNumber=10  BitShiftDirection=Left
  Md12 : ArithShift  BitShiftNumber=11  BitShiftDirection=Left
  Md13 : ArithShift  BitShiftNumber=12  BitShiftDirection=Left
  Md14 : ArithShift  BitShiftNumber=13  BitShiftDirection=Left
  Md15 : ArithShift  BitShiftNumber=14  BitShiftDirection=Left
  Md16 : ArithShift  BitShiftNumber=15  BitShiftDirection=Left
  Md17 : ArithShift  BitShiftNumber=16  BitShiftDirection=Left
  Md18 : ArithShift  BitShiftNumber=17  BitShiftDirection=Left
  Md19 : ArithShift  BitShiftNumber=18  BitShiftDirection=Left
  Md2 : ArithShift  BitShiftNumber=1  BitShiftDirection=Left
  Md20 : ArithShift  BitShiftNumber=19  BitShiftDirection=Left
  Md21 : ArithShift  BitShiftNumber=20  BitShiftDirection=Left
  Md22 : ArithShift  BitShiftNumber=21  BitShiftDirection=Left
  Md23 : ArithShift  BitShiftNumber=22  BitShiftDirection=Left
  Md24 : ArithShift  BitShiftNumber=23  BitShiftDirection=Left
  Md25 : ArithShift  BitShiftNumber=24  BitShiftDirection=Left
  Md26 : ArithShift  BitShiftNumber=25  BitShiftDirection=Left
  Md27 : ArithShift  BitShiftNumber=26  BitShiftDirection=Left
  Md28 : ArithShift  BitShiftNumber=27  BitShiftDirection=Left
  Md29 : ArithShift  BitShiftNumber=28  BitShiftDirection=Left
  Md3 : ArithShift  BitShiftNumber=2  BitShiftDirection=Left
  Md30 : ArithShift  BitShiftNumber=29  BitShiftDirection=Left
  Md31 : ArithShift  BitShiftNumber=30  BitShiftDirection=Left
  Md32 : ArithShift  BitShiftNumber=31  BitShiftDirection=Left
  Md4 : ArithShift  BitShiftNumber=3  BitShiftDirection=Left
  Md5 : ArithShift  BitShiftNumber=4  BitShiftDirection=Left
  Md6 : ArithShift  BitShiftNumber=5  BitShiftDirection=Left
  Md7 : ArithShift  BitShiftNumber=6  BitShiftDirection=Left
  Md8 : ArithShift  BitShiftNumber=7  BitShiftDirection=Left
  Md9 : ArithShift  BitShiftNumber=8  BitShiftDirection=Left
  MdXXHolder : Outport  VectorParamsAs1DForOutWhenUnconnected=off
  wires:
  Md30HoldReq/1 -> Data Type Conversion30/1
  Md3/1 -> Bitwise Operator1/3
  Data Type Conversion9/1 -> Md9/1
  Md5HoldReq/1 -> Data Type Conversion5/1
  Md13HoldReq/1 -> Data Type Conversion13/1
  Data Type Conversion32/1 -> Md32/1
  Md15HoldReq/1 -> Data Type Conversion15/1
  Data Type Conversion8/1 -> Md8/1
  Data Type Conversion3/1 -> Md3/1
  Md7HoldReq/1 -> Data Type Conversion7/1
  Md12HoldReq/1 -> Data Type Conversion12/1
  Data Type Conversion21/1 -> Md21/1
  Data Type Conversion12/1 -> Md12/1
  Md10HoldReq/1 -> Data Type Conversion10/1
  Md5/1 -> Bitwise Operator1/5
  Md14/1 -> Bitwise Operator1/14
  Md1/1 -> Bitwise Operator1/1
  Md9HoldReq/1 -> Data Type Conversion9/1
  Data Type Conversion27/1 -> Md27/1
  Data Type Conversion15/1 -> Md15/1
  Md29/1 -> Bitwise Operator1/29
  Md23/1 -> Bitwise Operator1/23
  Data Type Conversion10/1 -> Md10/1
  Md12/1 -> Bitwise Operator1/12
  Md31HoldReq/1 -> Data Type Conversion31/1
  Data Type Conversion22/1 -> Md22/1
  Bitwise Operator1/1 -> MdXXHolder/1
  Data Type Conversion31/1 -> Md31/1
  Md4/1 -> Bitwise Operator1/4
  Md27/1 -> Bitwise Operator1/27
  Data Type Conversion18/1 -> Md18/1
  Md9/1 -> Bitwise Operator1/9
  Md3HoldReq/1 -> Data Type Conversion3/1
  Data Type Conversion25/1 -> Md25/1
  Md14HoldReq/1 -> Data Type Conversion14/1
  Md27HoldReq/1 -> Data Type Conversion27/1
  Md4HoldReq/1 -> Data Type Conversion4/1
  Md7/1 -> Bitwise Operator1/7
  Md18HoldReq/1 -> Data Type Conversion18/1
  Md8/1 -> Bitwise Operator1/8
  Data Type Conversion7/1 -> Md7/1
  Data Type Conversion26/1 -> Md26/1
  Md17/1 -> Bitwise Operator1/17
  Data Type Conversion4/1 -> Md4/1
  Md18/1 -> Bitwise Operator1/18
  Md22HoldReq/1 -> Data Type Conversion22/1
  Md13/1 -> Bitwise Operator1/13
  Md2HoldReq/1 -> Data Type Conversion2/1
  Data Type Conversion2/1 -> Md2/1
  Md1HoldReq/1 -> Data Type Conversion1/1
  Data Type Conversion24/1 -> Md24/1
  Data Type Conversion13/1 -> Md13/1
  Md24HoldReq/1 -> Data Type Conversion24/1
  Data Type Conversion14/1 -> Md14/1
  Md22/1 -> Bitwise Operator1/22
  Data Type Conversion30/1 -> Md30/1
  Md32HoldReq/1 -> Data Type Conversion32/1
  Data Type Conversion5/1 -> Md5/1
  Md20HoldReq/1 -> Data Type Conversion20/1
  Md10/1 -> Bitwise Operator1/10
  Md11/1 -> Bitwise Operator1/11
  Data Type Conversion20/1 -> Md20/1
  Md21HoldReq/1 -> Data Type Conversion21/1
  Data Type Conversion23/1 -> Md23/1
  Md23HoldReq/1 -> Data Type Conversion23/1
  Md25HoldReq/1 -> Data Type Conversion25/1
  Data Type Conversion17/1 -> Md17/1
  Md17HoldReq/1 -> Data Type Conversion17/1
  Md6/1 -> Bitwise Operator1/6
  Md16/1 -> Bitwise Operator1/16
  Md15/1 -> Bitwise Operator1/15
  Md19/1 -> Bitwise Operator1/19
  Md6HoldReq/1 -> Data Type Conversion6/1
  Data Type Conversion19/1 -> Md19/1
  Md20/1 -> Bitwise Operator1/20
  Md21/1 -> Bitwise Operator1/21
  Md24/1 -> Bitwise Operator1/24
  Md25/1 -> Bitwise Operator1/25
  Md26/1 -> Bitwise Operator1/26
  Md28/1 -> Bitwise Operator1/28
  Md30/1 -> Bitwise Operator1/30
  Md31/1 -> Bitwise Operator1/31
  Md32/1 -> Bitwise Operator1/32
  Md2/1 -> Bitwise Operator1/2
  Md11HoldReq/1 -> Data Type Conversion11/1
  Data Type Conversion11/1 -> Md11/1
  Data Type Conversion6/1 -> Md6/1
  Md28HoldReq/1 -> Data Type Conversion28/1
  Data Type Conversion28/1 -> Md28/1
  Md16HoldReq/1 -> Data Type Conversion16/1
  Data Type Conversion16/1 -> Md16/1
  Md26HoldReq/1 -> Data Type Conversion26/1
  Md19HoldReq/1 -> Data Type Conversion19/1
  Data Type Conversion1/1 -> Md1/1
  Md8HoldReq/1 -> Data Type Conversion8/1
  Data Type Conversion29/1 -> Md29/1
  Md29HoldReq/1 -> Data Type Conversion29/1

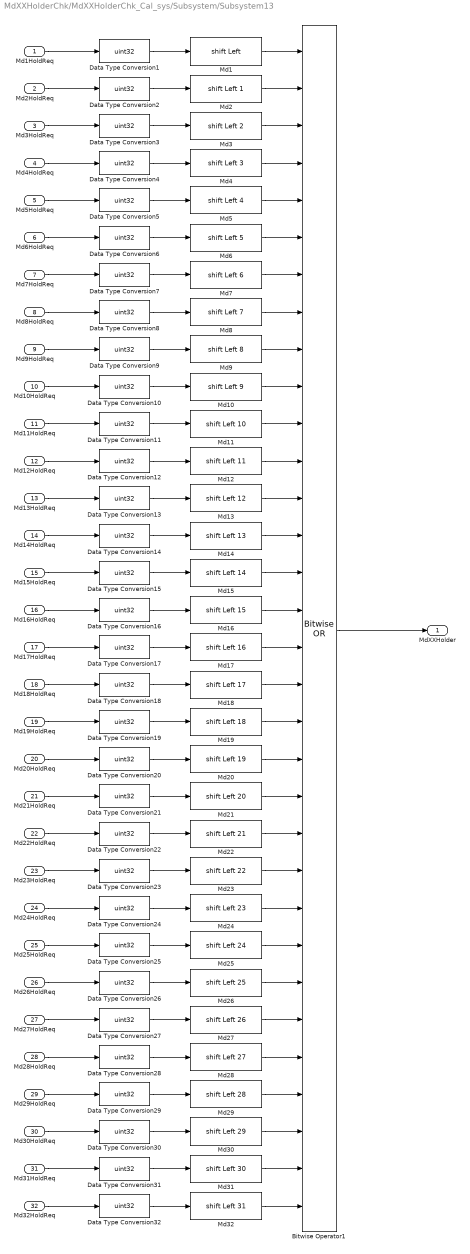
== system MdXXHolderChk/MdXXHolderChk_Cal_sys/Subsystem/Subsystem13 ==
  Md1HoldReq : Inport
  Md2HoldReq : Inport  Port=2
  Md3HoldReq : Inport  Port=3
  Md4HoldReq : Inport  Port=4
  Md5HoldReq : Inport  Port=5
  Md6HoldReq : Inport  Port=6
  Md7HoldReq : Inport  Port=7
  Md8HoldReq : Inport  Port=8
  Md9HoldReq : Inport  Port=9
  Md10HoldReq : Inport  Port=10
  Md11HoldReq : Inport  Port=11
  Md12HoldReq : Inport  Port=12
  Md13HoldReq : Inport  Port=13
  Md14HoldReq : Inport  Port=14
  Md15HoldReq : Inport  Port=15
  Md16HoldReq : Inport  Port=16
  Md17HoldReq : Inport  Port=17
  Md18HoldReq : Inport  Port=18
  Md19HoldReq : Inport  Port=19
  Md20HoldReq : Inport  Port=20
  Md21HoldReq : Inport  Port=21
  Md22HoldReq : Inport  Port=22
  Md23HoldReq : Inport  Port=23
  Md24HoldReq : Inport  Port=24
  Md25HoldReq : Inport  Port=25
  Md26HoldReq : Inport  Port=26
  Md27HoldReq : Inport  Port=27
  Md28HoldReq : Inport  Port=28
  Md29HoldReq : Inport  Port=29
  Md30HoldReq : Inport  Port=30
  Md31HoldReq : Inport  Port=31
  Md32HoldReq : Inport  Port=32
  Bitwise Operator1 : simulink/Logic and Bit Operations/Bitwise Operator  logicop=OR  UseBitMask=off  NumInputPorts=32  BitMask=bin2dec('11011001')  BitMaskRealWorld=Stored Integer
  Data Type Conversion{1..32} (32 alike) : DataTypeConversion  OutDataTypeStr=uint32  SaturateOnIntegerOverflow=off  RndMeth=Floor
  Md1 : ArithShift  BitShiftDirection=Left
  Md10 : ArithShift  BitShiftNumber=9  BitShiftDirection=Left
  Md11 : ArithShift  BitShiftNumber=10  BitShiftDirection=Left
  Md12 : ArithShift  BitShiftNumber=11  BitShiftDirection=Left
  Md13 : ArithShift  BitShiftNumber=12  BitShiftDirection=Left
  Md14 : ArithShift  BitShiftNumber=13  BitShiftDirection=Left
  Md15 : ArithShift  BitShiftNumber=14  BitShiftDirection=Left
  Md16 : ArithShift  BitShiftNumber=15  BitShiftDirection=Left
  Md17 : ArithShift  BitShiftNumber=16  BitShiftDirection=Left
  Md18 : ArithShift  BitShiftNumber=17  BitShiftDirection=Left
  Md19 : ArithShift  BitShiftNumber=18  BitShiftDirection=Left
  Md2 : ArithShift  BitShiftNumber=1  BitShiftDirection=Left
  Md20 : ArithShift  BitShiftNumber=19  BitShiftDirection=Left
  Md21 : ArithShift  BitShiftNumber=20  BitShiftDirection=Left
  Md22 : ArithShift  BitShiftNumber=21  BitShiftDirection=Left
  Md23 : ArithShift  BitShiftNumber=22  BitShiftDirection=Left
  Md24 : ArithShift  BitShiftNumber=23  BitShiftDirection=Left
  Md25 : ArithShift  BitShiftNumber=24  BitShiftDirection=Left
  Md26 : ArithShift  BitShiftNumber=25  BitShiftDirection=Left
  Md27 : ArithShift  BitShiftNumber=26  BitShiftDirection=Left
  Md28 : ArithShift  BitShiftNumber=27  BitShiftDirection=Left
  Md29 : ArithShift  BitShiftNumber=28  BitShiftDirection=Left
  Md3 : ArithShift  BitShiftNumber=2  BitShiftDirection=Left
  Md30 : ArithShift  BitShiftNumber=29  BitShiftDirection=Left
  Md31 : ArithShift  BitShiftNumber=30  BitShiftDirection=Left
  Md32 : ArithShift  BitShiftNumber=31  BitShiftDirection=Left
  Md4 : ArithShift  BitShiftNumber=3  BitShiftDirection=Left
  Md5 : ArithShift  BitShiftNumber=4  BitShiftDirection=Left
  Md6 : ArithShift  BitShiftNumber=5  BitShiftDirection=Left
  Md7 : ArithShift  BitShiftNumber=6  BitShiftDirection=Left
  Md8 : ArithShift  BitShiftNumber=7  BitShiftDirection=Left
  Md9 : ArithShift  BitShiftNumber=8  BitShiftDirection=Left
  MdXXHolder : Outport  VectorParamsAs1DForOutWhenUnconnected=off
  wires:
  Md30HoldReq/1 -> Data Type Conversion30/1
  Md3/1 -> Bitwise Operator1/3
  Data Type Conversion9/1 -> Md9/1
  Md5HoldReq/1 -> Data Type Conversion5/1
  Md13HoldReq/1 -> Data Type Conversion13/1
  Data Type Conversion32/1 -> Md32/1
  Md15HoldReq/1 -> Data Type Conversion15/1
  Data Type Conversion8/1 -> Md8/1
  Data Type Conversion3/1 -> Md3/1
  Md7HoldReq/1 -> Data Type Conversion7/1
  Md12HoldReq/1 -> Data Type Conversion12/1
  Data Type Conversion21/1 -> Md21/1
  Data Type Conversion12/1 -> Md12/1
  Md10HoldReq/1 -> Data Type Conversion10/1
  Md5/1 -> Bitwise Operator1/5
  Md14/1 -> Bitwise Operator1/14
  Md1/1 -> Bitwise Operator1/1
  Md9HoldReq/1 -> Data Type Conversion9/1
  Data Type Conversion27/1 -> Md27/1
  Data Type Conversion15/1 -> Md15/1
  Md29/1 -> Bitwise Operator1/29
  Md23/1 -> Bitwise Operator1/23
  Data Type Conversion10/1 -> Md10/1
  Md12/1 -> Bitwise Operator1/12
  Md31HoldReq/1 -> Data Type Conversion31/1
  Data Type Conversion22/1 -> Md22/1
  Bitwise Operator1/1 -> MdXXHolder/1
  Data Type Conversion31/1 -> Md31/1
  Md4/1 -> Bitwise Operator1/4
  Md27/1 -> Bitwise Operator1/27
  Data Type Conversion18/1 -> Md18/1
  Md9/1 -> Bitwise Operator1/9
  Md3HoldReq/1 -> Data Type Conversion3/1
  Data Type Conversion25/1 -> Md25/1
  Md14HoldReq/1 -> Data Type Conversion14/1
  Md27HoldReq/1 -> Data Type Conversion27/1
  Md4HoldReq/1 -> Data Type Conversion4/1
  Md7/1 -> Bitwise Operator1/7
  Md18HoldReq/1 -> Data Type Conversion18/1
  Md8/1 -> Bitwise Operator1/8
  Data Type Conversion7/1 -> Md7/1
  Data Type Conversion26/1 -> Md26/1
  Md17/1 -> Bitwise Operator1/17
  Data Type Conversion4/1 -> Md4/1
  Md18/1 -> Bitwise Operator1/18
  Md22HoldReq/1 -> Data Type Conversion22/1
  Md13/1 -> Bitwise Operator1/13
  Md2HoldReq/1 -> Data Type Conversion2/1
  Data Type Conversion2/1 -> Md2/1
  Md1HoldReq/1 -> Data Type Conversion1/1
  Data Type Conversion24/1 -> Md24/1
  Data Type Conversion13/1 -> Md13/1
  Md24HoldReq/1 -> Data Type Conversion24/1
  Data Type Conversion14/1 -> Md14/1
  Md22/1 -> Bitwise Operator1/22
  Data Type Conversion30/1 -> Md30/1
  Md32HoldReq/1 -> Data Type Conversion32/1
  Data Type Conversion5/1 -> Md5/1
  Md20HoldReq/1 -> Data Type Conversion20/1
  Md10/1 -> Bitwise Operator1/10
  Md11/1 -> Bitwise Operator1/11
  Data Type Conversion20/1 -> Md20/1
  Md21HoldReq/1 -> Data Type Conversion21/1
  Data Type Conversion23/1 -> Md23/1
  Md23HoldReq/1 -> Data Type Conversion23/1
  Md25HoldReq/1 -> Data Type Conversion25/1
  Data Type Conversion17/1 -> Md17/1
  Md17HoldReq/1 -> Data Type Conversion17/1
  Md6/1 -> Bitwise Operator1/6
  Md16/1 -> Bitwise Operator1/16
  Md15/1 -> Bitwise Operator1/15
  Md19/1 -> Bitwise Operator1/19
  Md6HoldReq/1 -> Data Type Conversion6/1
  Data Type Conversion19/1 -> Md19/1
  Md20/1 -> Bitwise Operator1/20
  Md21/1 -> Bitwise Operator1/21
  Md24/1 -> Bitwise Operator1/24
  Md25/1 -> Bitwise Operator1/25
  Md26/1 -> Bitwise Operator1/26
  Md28/1 -> Bitwise Operator1/28
  Md30/1 -> Bitwise Operator1/30
  Md31/1 -> Bitwise Operator1/31
  Md32/1 -> Bitwise Operator1/32
  Md2/1 -> Bitwise Operator1/2
  Md11HoldReq/1 -> Data Type Conversion11/1
  Data Type Conversion11/1 -> Md11/1
  Data Type Conversion6/1 -> Md6/1
  Md28HoldReq/1 -> Data Type Conversion28/1
  Data Type Conversion28/1 -> Md28/1
  Md16HoldReq/1 -> Data Type Conversion16/1
  Data Type Conversion16/1 -> Md16/1
  Md26HoldReq/1 -> Data Type Conversion26/1
  Md19HoldReq/1 -> Data Type Conversion19/1
  Data Type Conversion1/1 -> Md1/1
  Md8HoldReq/1 -> Data Type Conversion8/1
  Data Type Conversion29/1 -> Md29/1
  Md29HoldReq/1 -> Data Type Conversion29/1

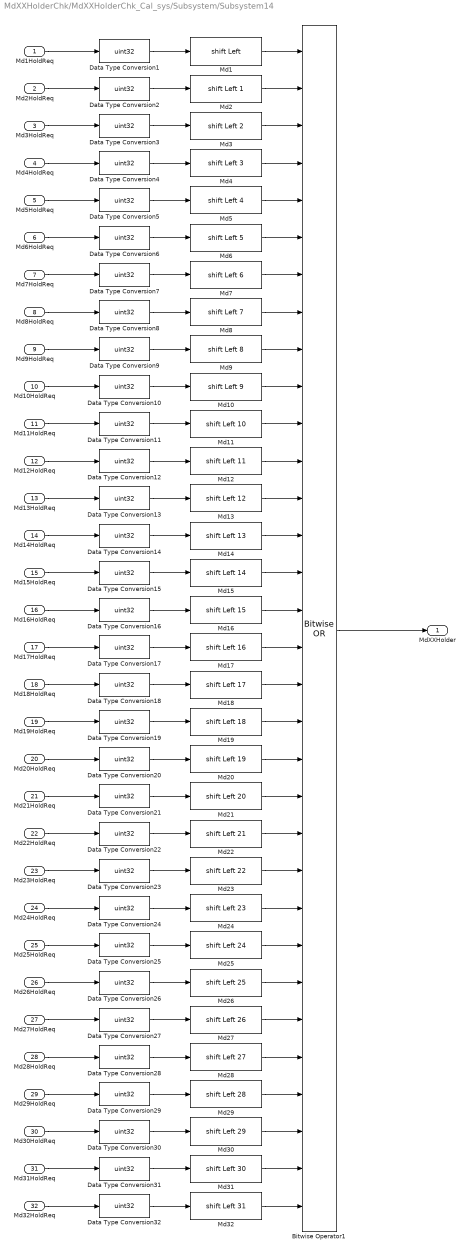
== system MdXXHolderChk/MdXXHolderChk_Cal_sys/Subsystem/Subsystem14 ==
  Md1HoldReq : Inport
  Md2HoldReq : Inport  Port=2
  Md3HoldReq : Inport  Port=3
  Md4HoldReq : Inport  Port=4
  Md5HoldReq : Inport  Port=5
  Md6HoldReq : Inport  Port=6
  Md7HoldReq : Inport  Port=7
  Md8HoldReq : Inport  Port=8
  Md9HoldReq : Inport  Port=9
  Md10HoldReq : Inport  Port=10
  Md11HoldReq : Inport  Port=11
  Md12HoldReq : Inport  Port=12
  Md13HoldReq : Inport  Port=13
  Md14HoldReq : Inport  Port=14
  Md15HoldReq : Inport  Port=15
  Md16HoldReq : Inport  Port=16
  Md17HoldReq : Inport  Port=17
  Md18HoldReq : Inport  Port=18
  Md19HoldReq : Inport  Port=19
  Md20HoldReq : Inport  Port=20
  Md21HoldReq : Inport  Port=21
  Md22HoldReq : Inport  Port=22
  Md23HoldReq : Inport  Port=23
  Md24HoldReq : Inport  Port=24
  Md25HoldReq : Inport  Port=25
  Md26HoldReq : Inport  Port=26
  Md27HoldReq : Inport  Port=27
  Md28HoldReq : Inport  Port=28
  Md29HoldReq : Inport  Port=29
  Md30HoldReq : Inport  Port=30
  Md31HoldReq : Inport  Port=31
  Md32HoldReq : Inport  Port=32
  Bitwise Operator1 : simulink/Logic and Bit Operations/Bitwise Operator  logicop=OR  UseBitMask=off  NumInputPorts=32  BitMask=bin2dec('11011001')  BitMaskRealWorld=Stored Integer
  Data Type Conversion{1..32} (32 alike) : DataTypeConversion  OutDataTypeStr=uint32  SaturateOnIntegerOverflow=off  RndMeth=Floor
  Md1 : ArithShift  BitShiftDirection=Left
  Md10 : ArithShift  BitShiftNumber=9  BitShiftDirection=Left
  Md11 : ArithShift  BitShiftNumber=10  BitShiftDirection=Left
  Md12 : ArithShift  BitShiftNumber=11  BitShiftDirection=Left
  Md13 : ArithShift  BitShiftNumber=12  BitShiftDirection=Left
  Md14 : ArithShift  BitShiftNumber=13  BitShiftDirection=Left
  Md15 : ArithShift  BitShiftNumber=14  BitShiftDirection=Left
  Md16 : ArithShift  BitShiftNumber=15  BitShiftDirection=Left
  Md17 : ArithShift  BitShiftNumber=16  BitShiftDirection=Left
  Md18 : ArithShift  BitShiftNumber=17  BitShiftDirection=Left
  Md19 : ArithShift  BitShiftNumber=18  BitShiftDirection=Left
  Md2 : ArithShift  BitShiftNumber=1  BitShiftDirection=Left
  Md20 : ArithShift  BitShiftNumber=19  BitShiftDirection=Left
  Md21 : ArithShift  BitShiftNumber=20  BitShiftDirection=Left
  Md22 : ArithShift  BitShiftNumber=21  BitShiftDirection=Left
  Md23 : ArithShift  BitShiftNumber=22  BitShiftDirection=Left
  Md24 : ArithShift  BitShiftNumber=23  BitShiftDirection=Left
  Md25 : ArithShift  BitShiftNumber=24  BitShiftDirection=Left
  Md26 : ArithShift  BitShiftNumber=25  BitShiftDirection=Left
  Md27 : ArithShift  BitShiftNumber=26  BitShiftDirection=Left
  Md28 : ArithShift  BitShiftNumber=27  BitShiftDirection=Left
  Md29 : ArithShift  BitShiftNumber=28  BitShiftDirection=Left
  Md3 : ArithShift  BitShiftNumber=2  BitShiftDirection=Left
  Md30 : ArithShift  BitShiftNumber=29  BitShiftDirection=Left
  Md31 : ArithShift  BitShiftNumber=30  BitShiftDirection=Left
  Md32 : ArithShift  BitShiftNumber=31  BitShiftDirection=Left
  Md4 : ArithShift  BitShiftNumber=3  BitShiftDirection=Left
  Md5 : ArithShift  BitShiftNumber=4  BitShiftDirection=Left
  Md6 : ArithShift  BitShiftNumber=5  BitShiftDirection=Left
  Md7 : ArithShift  BitShiftNumber=6  BitShiftDirection=Left
  Md8 : ArithShift  BitShiftNumber=7  BitShiftDirection=Left
  Md9 : ArithShift  BitShiftNumber=8  BitShiftDirection=Left
  MdXXHolder : Outport  VectorParamsAs1DForOutWhenUnconnected=off
  wires:
  Md30HoldReq/1 -> Data Type Conversion30/1
  Md3/1 -> Bitwise Operator1/3
  Data Type Conversion9/1 -> Md9/1
  Md5HoldReq/1 -> Data Type Conversion5/1
  Md13HoldReq/1 -> Data Type Conversion13/1
  Data Type Conversion32/1 -> Md32/1
  Md15HoldReq/1 -> Data Type Conversion15/1
  Data Type Conversion8/1 -> Md8/1
  Data Type Conversion3/1 -> Md3/1
  Md7HoldReq/1 -> Data Type Conversion7/1
  Md12HoldReq/1 -> Data Type Conversion12/1
  Data Type Conversion21/1 -> Md21/1
  Data Type Conversion12/1 -> Md12/1
  Md10HoldReq/1 -> Data Type Conversion10/1
  Md5/1 -> Bitwise Operator1/5
  Md14/1 -> Bitwise Operator1/14
  Md1/1 -> Bitwise Operator1/1
  Md9HoldReq/1 -> Data Type Conversion9/1
  Data Type Conversion27/1 -> Md27/1
  Data Type Conversion15/1 -> Md15/1
  Md29/1 -> Bitwise Operator1/29
  Md23/1 -> Bitwise Operator1/23
  Data Type Conversion10/1 -> Md10/1
  Md12/1 -> Bitwise Operator1/12
  Md31HoldReq/1 -> Data Type Conversion31/1
  Data Type Conversion22/1 -> Md22/1
  Bitwise Operator1/1 -> MdXXHolder/1
  Data Type Conversion31/1 -> Md31/1
  Md4/1 -> Bitwise Operator1/4
  Md27/1 -> Bitwise Operator1/27
  Data Type Conversion18/1 -> Md18/1
  Md9/1 -> Bitwise Operator1/9
  Md3HoldReq/1 -> Data Type Conversion3/1
  Data Type Conversion25/1 -> Md25/1
  Md14HoldReq/1 -> Data Type Conversion14/1
  Md27HoldReq/1 -> Data Type Conversion27/1
  Md4HoldReq/1 -> Data Type Conversion4/1
  Md7/1 -> Bitwise Operator1/7
  Md18HoldReq/1 -> Data Type Conversion18/1
  Md8/1 -> Bitwise Operator1/8
  Data Type Conversion7/1 -> Md7/1
  Data Type Conversion26/1 -> Md26/1
  Md17/1 -> Bitwise Operator1/17
  Data Type Conversion4/1 -> Md4/1
  Md18/1 -> Bitwise Operator1/18
  Md22HoldReq/1 -> Data Type Conversion22/1
  Md13/1 -> Bitwise Operator1/13
  Md2HoldReq/1 -> Data Type Conversion2/1
  Data Type Conversion2/1 -> Md2/1
  Md1HoldReq/1 -> Data Type Conversion1/1
  Data Type Conversion24/1 -> Md24/1
  Data Type Conversion13/1 -> Md13/1
  Md24HoldReq/1 -> Data Type Conversion24/1
  Data Type Conversion14/1 -> Md14/1
  Md22/1 -> Bitwise Operator1/22
  Data Type Conversion30/1 -> Md30/1
  Md32HoldReq/1 -> Data Type Conversion32/1
  Data Type Conversion5/1 -> Md5/1
  Md20HoldReq/1 -> Data Type Conversion20/1
  Md10/1 -> Bitwise Operator1/10
  Md11/1 -> Bitwise Operator1/11
  Data Type Conversion20/1 -> Md20/1
  Md21HoldReq/1 -> Data Type Conversion21/1
  Data Type Conversion23/1 -> Md23/1
  Md23HoldReq/1 -> Data Type Conversion23/1
  Md25HoldReq/1 -> Data Type Conversion25/1
  Data Type Conversion17/1 -> Md17/1
  Md17HoldReq/1 -> Data Type Conversion17/1
  Md6/1 -> Bitwise Operator1/6
  Md16/1 -> Bitwise Operator1/16
  Md15/1 -> Bitwise Operator1/15
  Md19/1 -> Bitwise Operator1/19
  Md6HoldReq/1 -> Data Type Conversion6/1
  Data Type Conversion19/1 -> Md19/1
  Md20/1 -> Bitwise Operator1/20
  Md21/1 -> Bitwise Operator1/21
  Md24/1 -> Bitwise Operator1/24
  Md25/1 -> Bitwise Operator1/25
  Md26/1 -> Bitwise Operator1/26
  Md28/1 -> Bitwise Operator1/28
  Md30/1 -> Bitwise Operator1/30
  Md31/1 -> Bitwise Operator1/31
  Md32/1 -> Bitwise Operator1/32
  Md2/1 -> Bitwise Operator1/2
  Md11HoldReq/1 -> Data Type Conversion11/1
  Data Type Conversion11/1 -> Md11/1
  Data Type Conversion6/1 -> Md6/1
  Md28HoldReq/1 -> Data Type Conversion28/1
  Data Type Conversion28/1 -> Md28/1
  Md16HoldReq/1 -> Data Type Conversion16/1
  Data Type Conversion16/1 -> Md16/1
  Md26HoldReq/1 -> Data Type Conversion26/1
  Md19HoldReq/1 -> Data Type Conversion19/1
  Data Type Conversion1/1 -> Md1/1
  Md8HoldReq/1 -> Data Type Conversion8/1
  Data Type Conversion29/1 -> Md29/1
  Md29HoldReq/1 -> Data Type Conversion29/1
